simulink model "SimulinkDiagram"  (R2024a)
settings: Solver=FixedStepAuto  StartTime=0.0  StopTime=2  FixedStep=1e-6  RelTol=1e-6  AbsTol=1e-3
values from neighbouring files (symbols this model uses):
  c = 0.154    [equations.m]
  f0 = m*0.3*9.8    (= 0.024696)    [equations.m]
  k = 2.5e4    (= 25000)    [equations.m]
  k_em = 15    [equations.m]
  L_e = 0.1    [equations.m]
  m = 8.4e-3    (= 0.0084)    [equations.m]
  R = 30000    [equations.m]
  R_e = 300    [equations.m]
  w = 275*2*pi    (= 1727.87595947)    [equations.m]
settings Model: Creator=iamme  LastModifiedBy=ma_as
settings SolverCC: AlgebraicLoopSolver=TrustRegion
settings DataIOCC: ReturnWorkspaceOutputs=off
settings DebuggingCC: UnconnectedInputMsg=warning  UnconnectedOutputMsg=warning  UnconnectedLineMsg=warning  ArithmeticOperatorsInVariantConditions=warning
settings ModelReferenceCC: EnableRefExpFcnMdlSchedulingChecks=on
settings SFSimCC: SimUseLocalCustomCode=off  CustomCodeUndefinedFunction=UseInterfaceOnly
settings RTWCC: RTWUseLocalCustomCode=off  GPUComputeCapability=3.5

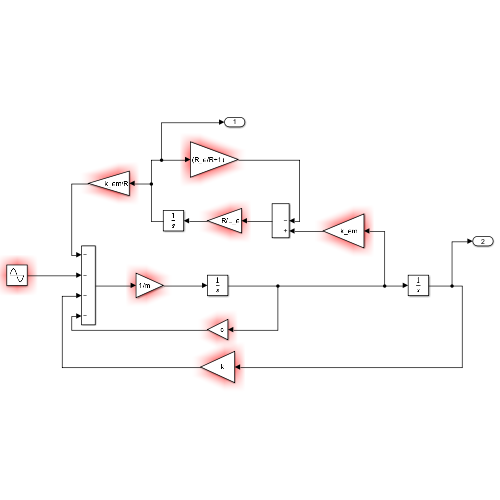
[thumbnail: Simulink's stored preview of the top-level diagram]
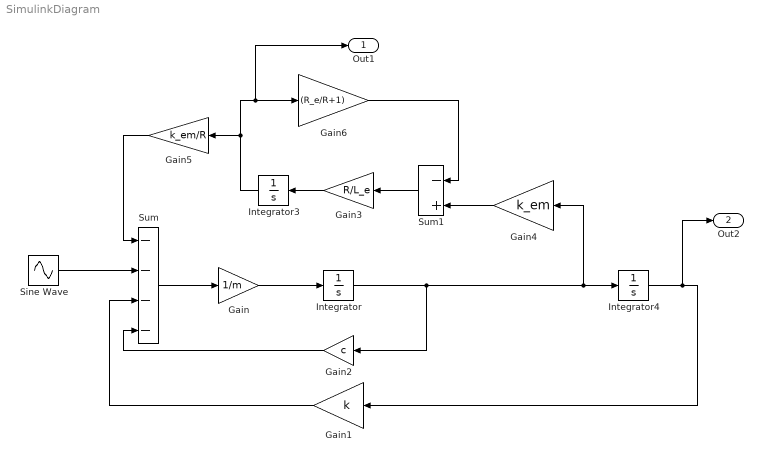
== system SimulinkDiagram ==
  Gain : Gain  Gain=1/m
  Gain1 : Gain  Gain=k
  Gain2 : Gain  Gain=c
  Gain3 : Gain  Gain=R/L_e
  Gain4 : Gain  Gain=k_em
  Gain5 : Gain  Gain=k_em/R
  Gain6 : Gain  Gain=(R_e/R+1)
  Integrator : Integrator
  Integrator3 : Integrator
  Integrator4 : Integrator
  Sine Wave : Sin  Amplitude=f0  Frequency=w  SampleTime=0
  Sum : Sum  Inputs=----
  Sum1 : Sum  Inputs=|-+
  Out1 : Outport  VectorParamsAs1DForOutWhenUnconnected=off
  Out2 : Outport  Port=2  VectorParamsAs1DForOutWhenUnconnected=off
  wires:
  Sum/1 -> Gain/1
  Gain/1 -> Integrator/1
  Integrator/1 -> Integrator4/1, Gain4/1, Gain2/1
  Gain2/1 -> Sum/4
  Gain1/1 -> Sum/3
  Integrator4/1 -> Out2/1, Gain1/1
  Gain4/1 -> Sum1/2
  Gain3/1 -> Integrator3/1
  Integrator3/1 -> Out1/1, Gain6/1, Gain5/1
  Gain5/1 -> Sum/1
  Gain6/1 -> Sum1/1
  Sine Wave/1 -> Sum/2
  Sum1/1 -> Gain3/1
